simulink model "skyhook_control"  (R2020b)
settings: Solver=VariableStepAuto  StartTime=0.0  StopTime=10.0  RelTol=1e-3
values from neighbouring files (symbols this model uses):
  K = lqr( A, B(:,2), Q, R )    [Active_suspension_open_loop_setup.m]
settings Model: Creator=admin  LastModifiedBy=admin

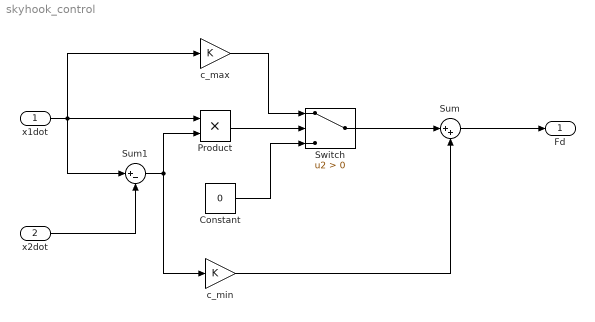
== system skyhook_control ==
  x1dot : Inport
  x2dot : Inport  Port=2
  Constant : Constant  Value=0
  Product : Product
  Sum : Sum  Inputs=|++
  Sum1 : Sum  Inputs=|+-
  Switch : Switch  Criteria=u2 > Threshold  ZeroCross=off
  c_max : Gain  Gain=K
  c_min : Gain  Gain=K
  Fd : Outport
  wires:
  x2dot/1 -> Sum1/2
  x1dot/1 -> c_max/1, Sum1/1, Product/1
  Sum1/1 -> Product/2, c_min/1
  Product/1 -> Switch/2
  Constant/1 -> Switch/3
  c_min/1 -> Sum/2
  Switch/1 -> Sum/1
  Sum/1 -> Fd/1
  c_max/1 -> Switch/1
